simulink model "Filter_Simulation"  (R2017a)
settings: Solver=FixedStepAuto  StartTime=0.0  StopTime=0.1  FixedStep=1e-6  RelTol=1e-3
StopFcn:
  | dlmwrite("TestData.csv", [round(filter_input.time*1000000), round(filter_input.data), round(filter_output.data)], 'precision', '%i')
values from neighbouring files (symbols this model uses):
  b = b*1024    [FIR_Filter_Design.m]
settings Model: Creator=Max  LastModifiedBy=Max

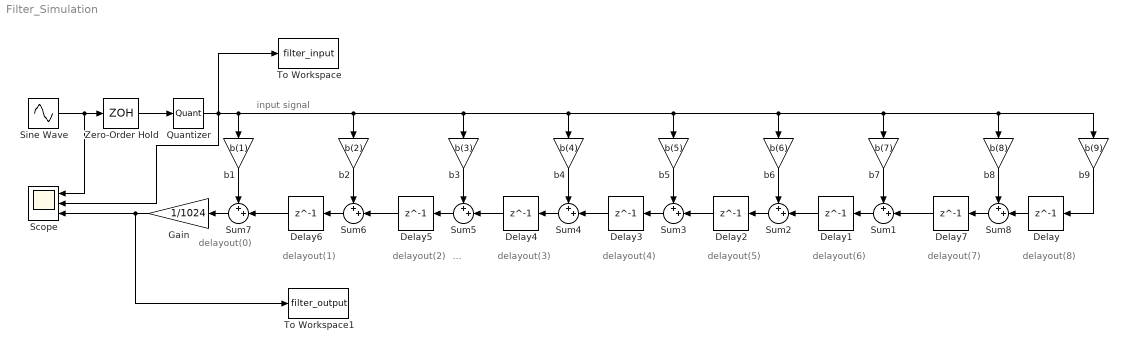
== system Filter_Simulation ==
  note: input signal
  note: delayout(8)
  note: ...
  note: delayout(7)
  note: delayout(6)
  note: delayout(5)
  note: delayout(4)
  note: delayout(3)
  note: delayout(2)
  note: delayout(1)
  note: delayout(0)
  Delay{,1..7} (8 alike) : Delay  DelayLength=1  InitialCondition=0
  Gain : Gain  Gain=1/1024
  Quantizer : Quantizer  QuantizationInterval=0.000244140625
  Scope : Scope  NumInputPorts=3
  Sine Wave : Sin  Amplitude=2047  Frequency=942  SampleTime=0
  Sum{1..8} (8 alike) : Sum  Inputs=++|
  To Workspace : ToWorkspace  VariableName=filter_input  SaveFormat=Timeseries  SampleTime=-1
  To Workspace1 : ToWorkspace  VariableName=filter_output  SaveFormat=Timeseries  SampleTime=-1
  Zero-Order Hold : ZeroOrderHold  SampleTime=1e-3
  b1 : Gain  Gain=b(1)
  b2 : Gain  Gain=b(2)
  b3 : Gain  Gain=b(3)
  b4 : Gain  Gain=b(4)
  b5 : Gain  Gain=b(5)
  b6 : Gain  Gain=b(6)
  b7 : Gain  Gain=b(7)
  b8 : Gain  Gain=b(8)
  b9 : Gain  Gain=b(9)
  wires:
  Sum1/1 -> Delay1/1
  Sum2/1 -> Delay2/1
  Sum3/1 -> Delay3/1
  Sum4/1 -> Delay4/1
  Sum5/1 -> Delay5/1
  Sum6/1 -> Delay6/1
  b7/1 -> Sum1/1
  b1/1 -> Sum7/1
  b2/1 -> Sum6/1
  b3/1 -> Sum5/1
  b4/1 -> Sum4/1
  b5/1 -> Sum3/1
  b6/1 -> Sum2/1
  b9/1 -> Delay/1
  Delay6/1 -> Sum7/2
  Delay5/1 -> Sum6/2
  Delay4/1 -> Sum5/2
  Delay3/1 -> Sum4/2
  Delay1/1 -> Sum2/2
  Sine Wave/1 -> Scope/1, Zero-Order Hold/1
  Delay2/1 -> Sum3/2
  Zero-Order Hold/1 -> Quantizer/1
  Quantizer/1 -> To Workspace/1, Scope/2, b8/1, b9/1, b7/1, b6/1, b5/1, b4/1, b3/1, b2/1, b1/1
  Sum7/1 -> Gain/1
  Sum8/1 -> Delay7/1
  b8/1 -> Sum8/1
  Delay7/1 -> Sum1/2
  Delay/1 -> Sum8/2
  Gain/1 -> To Workspace1/1, Scope/3
